simulink model "cylinder_buoy_1D"  (R2025b)
settings: Solver=FixedStepAuto  StartTime=0.0  StopTime=inf  FixedStep=0.0001  RelTol=1e-3
undefined symbols (not defined in the file): DiscIntNeverNeededParam
libraries: simulink x3, SG_DLE_position_control_module_hose_pump x1, servo_valve_pressure_control_module x1
settings Model: Creator=cmmcguir  LastModifiedBy=cmmcguir
settings SolverCC: ConcurrentTasks=on  PositivePriorityOrder=on
settings OptimizationCC: BlockReduction=off  OptimizeBlockIOStorage=off
settings DebuggingCC: TasksWithSamePriorityMsg=none
settings HardwareCC: ProdBitPerLong=64.0  ProdLongLongMode=on  ProdHWDeviceType=Intel->x86-64 (Linux 64)
settings RTWCC: SystemTargetFile=speedgoat.tlc  TemplateMakefile=slrealtime_default_tmf  Toolchain=Simulink Real-Time Toolchain  BuildConfiguration=Faster Runs  CodeExecutionProfiling=on  TargetLang=C++  Description=Speedgoat Real-Time Target Machine
settings SimulinkRealTimeTargetCC: SLRTFileLogMaxRuns=3.0  ExtModeMaxTrigDuration=10.0  ExtModeStaticAllocSize=1000000.0  ExtModeTransport=0.0  MultiwordLength=2048.0  DynamicStringBufferSize=256.0  PreserveMATLABNamespacesInGeneratedCode=on  SubcomponentCodeInterfacePackaging=Reusable function  MATLABClassNameForMDSCustomization=Simulink.SoftwareTarget.GRTCustomization  InstructionSetFMA=off  LogToMDFFile=off

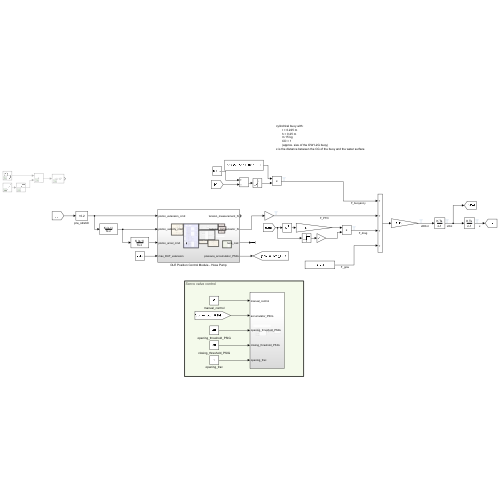
[thumbnail: Simulink's stored preview of the top-level diagram]
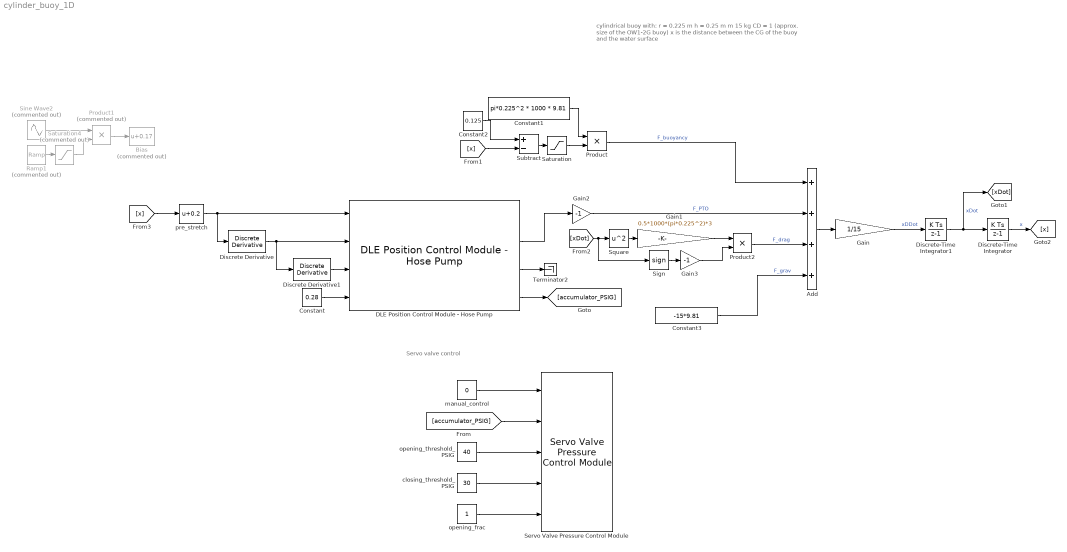
== system cylinder_buoy_1D ==
  note: cylindrical buoy with:
      | 	r = 0.225 m
      | 	h = 0.25 m
      | 	m 15 kg
      | 	CD = 1
      | 	(approx. size of the OW1-2G buoy)
      | x is the distance between the CG of the buoy and the water surface
  note: Servo valve control
  Add : Sum  Inputs=++++
  Bias : Bias  Commented=on  Bias=0.17  SaturateOnIntegerOverflow=off
  Constant : Constant  Value=0.28
  Constant1 : Constant  Value=pi*0.225^2 * 1000 * 9.81
  Constant2 : Constant  Value=0.125
  Constant3 : Constant  Value=-15*9.81
  DLE Position Control Module - Hose Pump : SG_DLE_position_control_module_hose_pump/DLE Position Control Module - Hose Pump  SystemSampleTime=-1  VariantActivationTime=update diagram  EmptyChoice=off  PassThrough=off  PassThroughVariantControl=(default)  EmptyChoiceVariantControl=(default)  AllowFlexibleInterface=on  Latency=0  AutoFrameSizeCalculation=off
  Discrete Derivative : simulink/Discrete/Discrete Derivative  gainval=1.0  ICPrevScaledInput=0.0  OutMin=[]  OutMax=[]  OutDataType=fixdt(1, 16)  OutScaling=2^-10  DoSatur=off
  Discrete Derivative1 : simulink/Discrete/Discrete Derivative  gainval=1.0  ICPrevScaledInput=0.0  OutMin=[]  OutMax=[]  OutDataType=fixdt(1, 16)  OutScaling=2^-10  DoSatur=off
  Discrete-Time Integrator : DiscreteIntegrator  SampleTime=-1  ICPrevOutput=DiscIntNeverNeededParam  ICPrevScaledInput=DiscIntNeverNeededParam
  Discrete-Time Integrator1 : DiscreteIntegrator  SampleTime=-1  ICPrevOutput=DiscIntNeverNeededParam  ICPrevScaledInput=DiscIntNeverNeededParam
  Gain : Gain  Gain=1/15
  Gain1 : Gain  Gain=0.5*1000*(pi*0.225^2)*3
  Gain2 : Gain  Gain=-1
  Gain3 : Gain  Gain=-1
  Product : Product
  Product1 : Product  Commented=on
  Product2 : Product
  Ramp1 : simulink/Sources/Ramp  Commented=on  slope=1/10  start=10  InitialOutput=0
  Saturation : Saturate  UpperLimit=0.25  LowerLimit=0
  Saturation4 : Saturate  Commented=on  UpperLimit=1  LowerLimit=0
  Servo Valve Pressure Control Module : servo_valve_pressure_control_module/Servo Valve Pressure Control Module  SystemSampleTime=-1  VariantActivationTime=update diagram  EmptyChoice=off  PassThrough=off  PassThroughVariantControl=(default)  EmptyChoiceVariantControl=(default)  AllowFlexibleInterface=on  Latency=0  AutoFrameSizeCalculation=off
  Sign : Signum
  Sine Wave2 : Sin  Commented=on  Amplitude=0.05  Frequency=2*pi/5  SampleTime=0.0001
  Square : Math  Operator=square
  Subtract : Sum  Inputs=+-
  Terminator2 : Terminator
  closing_threshold_PSIG : Constant  Value=30
  manual_control : Constant  Value=0  SampleTime=0.0001
  opening_frac : Constant
  opening_threshold_PSIG : Constant  Value=40
  pre_stretch : Bias  Bias=0.2  SaturateOnIntegerOverflow=off
  wires:
  Constant/1 -> DLE Position Control Module - Hose Pump/4
  Sine Wave2/1 -> Product1/1
  Product1/1 -> Bias/1
  Saturation4/1 -> Product1/2
  Discrete Derivative1/1 -> DLE Position Control Module - Hose Pump/3
  Ramp1/1 -> Saturation4/1
  pre_stretch/1 -> DLE Position Control Module - Hose Pump/1, Discrete Derivative/1
  Discrete Derivative/1 -> DLE Position Control Module - Hose Pump/2, Discrete Derivative1/1
  opening_frac/1 -> Servo Valve Pressure Control Module/5
  opening_threshold_PSIG/1 -> Servo Valve Pressure Control Module/3
  manual_control/1 -> Servo Valve Pressure Control Module/1
  closing_threshold_PSIG/1 -> Servo Valve Pressure Control Module/4
  [accumulator_PSIG] -> Servo Valve Pressure Control Module/2
  DLE Position Control Module - Hose Pump/2 -> Gain2/1
  DLE Position Control Module - Hose Pump/3 -> Terminator2/1
  DLE Position Control Module - Hose Pump/4 -> [accumulator_PSIG]
  Gain/1 -> Discrete-Time Integrator1/1  "xDDot"
  Add/1 -> Gain/1
  [x] -> Subtract/2
  Constant2/1 -> Subtract/1
  Subtract/1 -> Saturation/1
  Saturation/1 -> Product/2
  Constant1/1 -> Product/1
  Product/1 -> Add/1  "F_buoyancy"
  [xDot] -> Sign/1, Square/1
  Square/1 -> Gain1/1
  Gain1/1 -> Product2/1
  Discrete-Time Integrator1/1 -> Discrete-Time Integrator/1, [xDot]  "xDot"
  Discrete-Time Integrator/1 -> [x]  "x"
  Constant3/1 -> Add/4  "F_grav"
  Gain2/1 -> Add/2  "F_PTO"
  Sign/1 -> Gain3/1
  Gain3/1 -> Product2/2
  Product2/1 -> Add/3  "F_drag"
  [x] -> pre_stretch/1
